simulink model "aufgabe1_nonlinear_reibung_c10_anfangsbedingung2"  (R2023b)
settings: Solver=VariableStepAuto  StartTime=0.0  StopTime=10.0  RelTol=1e-3
settings Model: Creator=serkan  LastModifiedBy=serkan

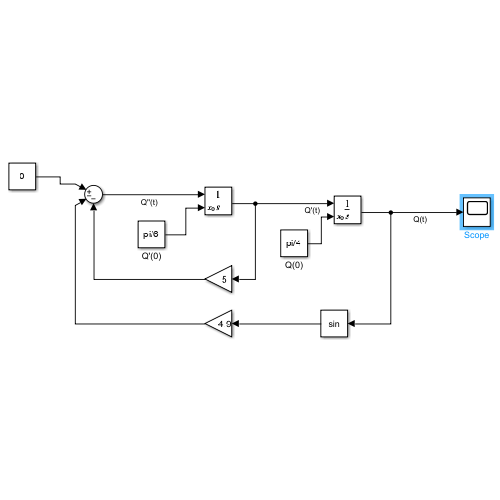
[thumbnail: Simulink's stored preview of the top-level diagram]
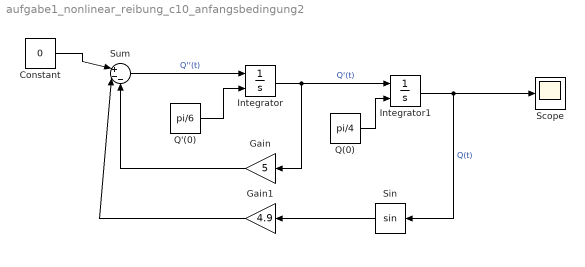
== system aufgabe1_nonlinear_reibung_c10_anfangsbedingung2 ==
  Constant : Constant  Value=0
  Gain : Gain  Gain=5
  Gain1 : Gain  Gain=4.9
  Integrator : Integrator  InitialConditionSource=external
  Integrator1 : Integrator  InitialConditionSource=external
  Q'(0) : Constant  Value=pi/6
  Q(0) : Constant  Value=pi/4
  Scope : Scope
  Sin : Trigonometry
  Sum : Sum  Inputs=|+--
  wires:
  Integrator1/1 -> Scope/1, Sin/1  "Q(t)"
  Sum/1 -> Integrator/1  "Q''(t)"
  Constant/1 -> Sum/1
  Integrator/1 -> Integrator1/1, Gain/1  "Q'(t)"
  Q(0)/1 -> Integrator1/2
  Gain1/1 -> Sum/2
  Gain/1 -> Sum/3
  Sin/1 -> Gain1/1
  Q'(0)/1 -> Integrator/2
